simulink model "prelookup_2d_lagrange_test_R2019a"  (R2019a)
settings: Solver=FixedStepDiscrete  StartTime=0.0  StopTime=1  FixedStep=1  RelTol=1e-3
Description:
  | 2-D Interpolation Using Prelookup (Linear Lagrange) test harness
settings Model: Creator=Administrator  LastModifiedBy=Administrator
settings DebuggingCC: UnconnectedInputMsg=none  UnconnectedOutputMsg=none  UnconnectedLineMsg=none
settings ModelReferenceCC: UpdateModelReferenceTargets=IfOutOfDate  EnableRefExpFcnMdlSchedulingChecks=off
settings RTWCC: Description=Generic Real-Time Target
settings ConfigComp: CovBoundaryAbsTol=1.0e-5

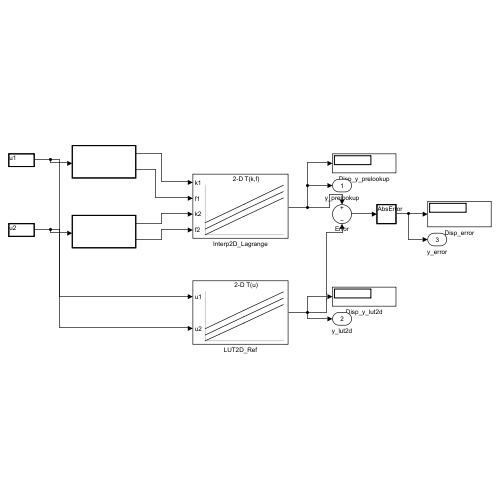
[thumbnail: Simulink's stored preview of the top-level diagram]
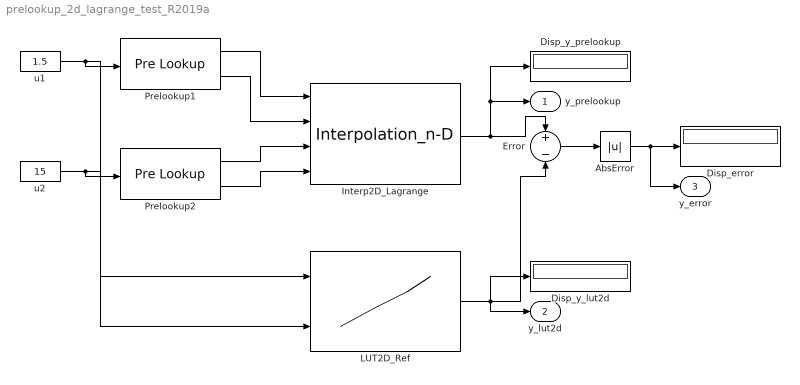
== system prelookup_2d_lagrange_test_R2019a ==
  AbsError : Abs
  Disp_error : Display
  Disp_y_lut2d : Display
  Disp_y_prelookup : Display
  Error : Sum  Inputs=+-
  Interp2D_Lagrange : Interpolation_n-D  Table=[100 200 300;400 500 600;700 800 900]  InterpMethod=Linear Lagrange  ExtrapMethod=Clip  InternalRulePriority=Speed
  LUT2D_Ref : Lookup_n-D  BreakpointsForDimension1=[1 2 3]  BreakpointsForDimension2=[10 20 30]  Table=[100 200 300;400 500 600;700 800 900]  InterpMethod=Linear Lagrange  ExtrapMethod=Clip  InternalRulePriority=Speed  RndMeth=Simplest  InputSameDT=on
  Prelookup1 : PreLookup  BreakpointsData=[1 2 3]
  Prelookup2 : PreLookup  BreakpointsData=[10 20 30]
  u1 : Constant  Value=1.5
  u2 : Constant  Value=15
  y_prelookup : Outport
  y_lut2d : Outport  Port=2
  y_error : Outport  Port=3
  wires:
  u1/1 -> Prelookup1/1, LUT2D_Ref/1
  u2/1 -> Prelookup2/1, LUT2D_Ref/2
  Prelookup1/1 -> Interp2D_Lagrange/1
  Prelookup1/2 -> Interp2D_Lagrange/2
  Prelookup2/1 -> Interp2D_Lagrange/3
  Prelookup2/2 -> Interp2D_Lagrange/4
  Interp2D_Lagrange/1 -> Disp_y_prelookup/1, y_prelookup/1, Error/1
  LUT2D_Ref/1 -> Error/2, Disp_y_lut2d/1, y_lut2d/1
  Error/1 -> AbsError/1
  AbsError/1 -> Disp_error/1, y_error/1
